simulink model "exp4"  (R2024a)
settings: Solver=VariableStepAuto  StartTime=0.0  StopTime=0.18  RelTol=1e-3
libraries: spsDetailedThyristorLib x4, spsVoltageMeasurementLib x2, spsACVoltageSourceLib x1, spsCurrentMeasurementLib x1, spsLinearTransformerLib x1, spsSeriesRLCBranchLib x1, sps_lib x1
settings Model: Creator=おもい  LastModifiedBy=おもい

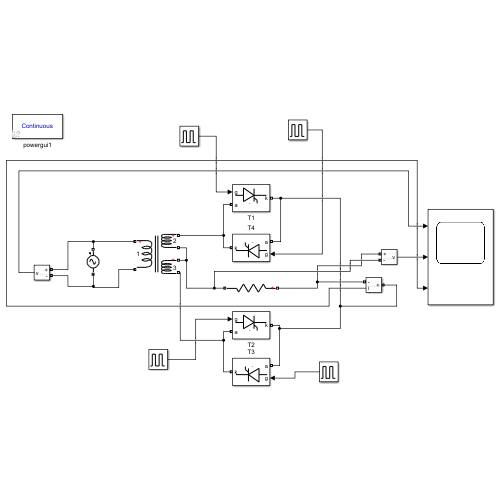
[thumbnail: Simulink's stored preview of the top-level diagram]
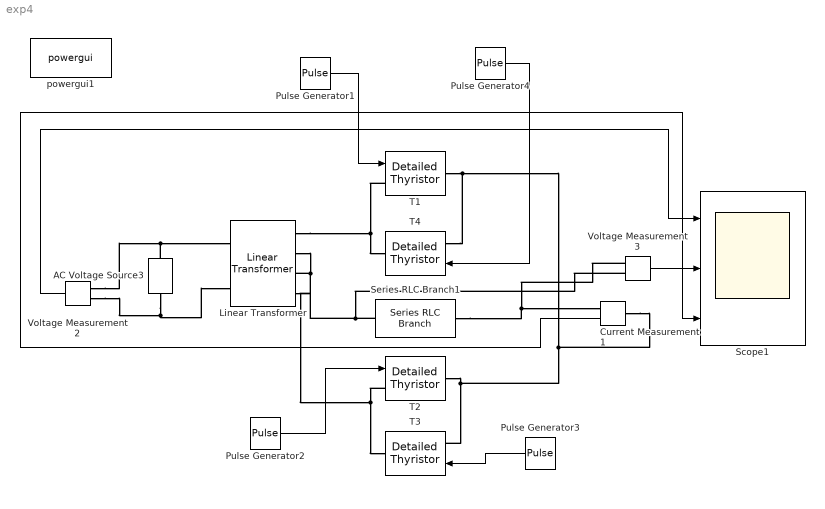
== system exp4 ==
  AC Voltage Source3 : spsACVoltageSourceLib/AC Voltage Source  Amplitude=200  Phase=0  Frequency=50  SampleTime=0  Measurements=None  BusType=swing  Pref=10e3  Qref=0  Qmin=-inf  Qmax=+inf
  Current Measurement1 : spsCurrentMeasurementLib/Current Measurement  PhasorSimulation=off  OutputType=Complex  PSBequivalent=0
  Linear Transformer : spsLinearTransformerLib/Linear Transformer  UNITS=pu  NominalPower=[ 250e6 50 ]  winding1="[ 630e3  0.002  0.08 ]"  winding2="[ 315e3  0.002  0.08 ]"  ThreeWindings=on  winding3=[ 315e3 0.002 0.08 ]  RmLm=[ 500 500 ]  Measurements=None  DataType=off
  Pulse Generator1 : DiscretePulseGenerator  PulseType=Time based  Amplitude=5  Period=0.06  PulseWidth=40
  Pulse Generator2 : DiscretePulseGenerator  PulseType=Time based  Amplitude=5  Period=0.06  PulseWidth=40  PhaseDelay=0.015
  Pulse Generator3 : DiscretePulseGenerator  PulseType=Time based  Amplitude=5  Period=0.06  PulseWidth=40  PhaseDelay=0.03
  Pulse Generator4 : DiscretePulseGenerator  PulseType=Time based  Amplitude=5  Period=0.06  PulseWidth=40  PhaseDelay=0.045
  Scope1 : Scope  NumInputPorts=3
  Series RLC Branch1 : spsSeriesRLCBranchLib/Series RLC Branch  LConnTagsString=__new0  RConnTagsString=__new0  BranchType=R  Resistance=50  Inductance=0.05  SetiL0=off  InitialCurrent=0  Capacitance=1e-6  Setx0=off  InitialVoltage=0  Measurements=None
  T{1..4} (4 alike) : spsDetailedThyristorLib/Detailed Thyristor  Ron=0.001  Lon=1e-3  Vf=0.8  IL=0.1  Tq=100e-6  IC=0  Rs=inf  Cs=inf  Measurements=off
      settings: LibrarySourceBlock=sps_lib/Power Electronics/Detailed Thyristor
  Voltage Measurement2 : spsVoltageMeasurementLib/Voltage Measurement  PhasorSimulation=off  OutputType=Complex  PSBequivalent=0
  Voltage Measurement3 : spsVoltageMeasurementLib/Voltage Measurement  PhasorSimulation=off  OutputType=Complex  PSBequivalent=0
  powergui1 : sps_lib/powergui  Priority=1  SimulationMode=Continuous  SampleTime=50e-6  frequency=60  Iterations=50  frequencyindice=50  Pbase=100e6  ErrMax=1e-4  UnitsV=kV  UnitsW=MW  buscounter=0  FunctionMessages=off  echomessages=off  EnableUseOfTLC=off  CurrentSourceSwitches=off  DisableSnubberDevices=off  DisableRonSwitches=off  DisableVfSwitches=off  DisplayEquations=off  AutomaticDiscreteSolvers=off  SolverType=Tustin/Backward Euler (TBE)  Interpol=off  ExternalGateDelay=off  methode=off  Ts=100  x0status=blocks  SPID=on  SwTol=0  HookPort=off  NonlinearTolerance=1e-4  nMaxIteration=100  ContinueOnMaxIteration=off  RestoreLinks=warning  ResistiveCurrentMeasurement=off  Frange=[0:2:500]  Ylog=off  Xlog=on  ShowGrid=off  save=off  variable=ZData  structure=0  ZoomFFT=off  StartTime=0.0  cycles=1  DisplayStyle=1  fundamental=60  FreqAxis=off  MaxFrequency=1000  frequencyindicesteady=1  RmsSteady=1  display=off
  wires:
  Voltage Measurement3/1 -> Scope1/2
  Pulse Generator1/1 -> T1/1
  Pulse Generator4/1 -> T4/1
  Pulse Generator2/1 -> T2/1
  Pulse Generator3/1 -> T3/1
  Current Measurement1/1 -> Scope1/3
  Voltage Measurement2/1 -> Scope1/1
  connections:
  AC Voltage Source3/RConn1 -- Linear Transformer/LConn1 -- Voltage Measurement2/LConn1
  AC Voltage Source3/LConn1 -- Voltage Measurement2/LConn2 -- Linear Transformer/LConn2
  T2/RConn1 -- T4/LConn1 -- T1/RConn1 -- Current Measurement1/LConn1 -- T3/LConn1
  T1/LConn1 -- Linear Transformer/RConn1 -- T4/RConn1
  T2/LConn1 -- Linear Transformer/RConn4 -- T3/RConn1
  Linear Transformer/RConn2 -- Voltage Measurement3/LConn2 -- Series RLC Branch1/RConn1 -- Linear Transformer/RConn3
  Series RLC Branch1/LConn1 -- Voltage Measurement3/LConn1 -- Current Measurement1/RConn1
